simulink model "ClosedLoop_sim"  (Simulink 9.2)
settings: Solver=VariableStepAuto  StartTime=0.0  StopTime=10.0  RelTol=1e-3
libraries: neural x305, simulink x1
(part 13 of 13)

== system ClosedLoop_sim/bigger_controller/Layer 4/Delays 1 ==
  "p{4}" : Inport  PortDimensions=100
      mask Display: e = 0.06;c1 = [120 230 180]/255;c2 = ([120 230 180]+0)/(256+128);c3 = ([120 230 180]+128)/(256+128);patch([0 1 1 0],[0 0 1 1],c1);patch([0 1 1 1-e 1-e 0+e],[0 0 1 1-e 0+e 0+e],c2);patch([0 0 1 1-e 0+e 0+e],[0 1 1 1-e 1-e 0+e],c3);plot([0 1 1 0 0],[0 0 1 1 0]);
  mux : Mux  Inputs=1
      mask Display: e = 0.06;c1 = [120 150 230]/255;c2 = ([120 150 230]+0)/383;c3 = ([120 150 230]+128)/383;patch([0 1 1 0],[0 0 1 1],c1);patch([0 1 1 1-e 1-e 0+e],[0 0 1 1-e 0+e 0+e],c2);patch([0 0 1 1-e 0+e 0+e],[0 1 1 1-e 1-e 0+e],c3);plot([0 1 1 0 0],[0 0 1 1 0]);disp('Mux')
  "pd{4,3}" : Outport
      mask Display: e = 0.06;c1 = [120 230 180]/255;c2 = ([120 230 180]+0)/(256+128);c3 = ([120 230 180]+128)/(256+128);patch([0 1 1 0],[0 0 1 1],c1);patch([0 1 1 1-e 1-e 0+e],[0 0 1 1-e 0+e 0+e],c2);patch([0 0 1 1-e 0+e 0+e],[0 1 1 1-e 1-e 0+e],c3);plot([0 1 1 0 0],[0 0 1 1 0]);
  wires:
  mux/1 -> "pd{4,3}"/1
  "p{4}"/1 -> mux/1

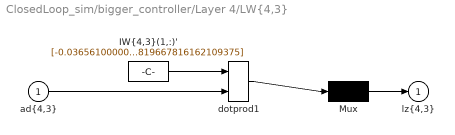
== system ClosedLoop_sim/bigger_controller/Layer 4/LW{4,3} ==
  "ad{4,3}" : Inport  PortDimensions=100
      mask Display: e = 0.06;c1 = [120 230 180]/255;c2 = ([120 230 180]+0)/(256+128);c3 = ([120 230 180]+128)/(256+128);patch([0 1 1 0],[0 0 1 1],c1);patch([0 1 1 1-e 1-e 0+e],[0 0 1 1-e 0+e 0+e],c2);patch([0 0 1 1-e 0+e 0+e],[0 1 1 1-e 1-e 0+e],c3);plot([0 1 1 0 0],[0 0 1 1 0]);
  "IW{4,3}(1,:)'" : Constant  Value=[-0.036561000000000003218314503783403779380023479461669921875;-0.09285100000000000297628588441511965356767177581787109375;-0.0752049999999999940758499406001647002995014190673828125;-0.01078299999999999918276483157342227059416472911834716796875;0.1605930000000000135162991909965057857334613800048828125;-0.06917700000000000237765362953723524697124958038330078125;0.311236000000000012644107982850982807576656341552734375;0.1429970000000000129869448528552311472594738006591796875;0.1426739999999999952695617366771330125629901885986328125;0.18814900000000001067945731847430579364299774169921875;0.14923100000000000253663756666355766355991363525390625;-0.1501159999999999994368948819101206026971340179443359375;0.06925199999999999411759432632607058621942996978759765625;-0.045718000000000001692423978738588630221784114837646484375;-0.0869270000000000042650327714000013656914234161376953125;0.0302669999999999987660981304316010209731757640838623046875;0.010054000000000000436539693282611551694571971893310546875;-0.083737000000000005872635711057228036224842071533203125;0.0338320000000000009610090501155355013906955718994140625;0.0203340000000000013791190411893694545142352581024169921875;-0.071068999999999993288923860745853744447231292724609375;-0.100376999999999994006572023863554932177066802978515625;0.039612000000000001376232461325344047509133815765380859375;0.054376000000000000722533144426051876507699489593505859375;0.1535060000000000035580427493187016807496547698974609375;-0.1376380000000000103366204484700574539601802825927734375;0.0712990000000000012647660696529783308506011962890625;-0.06631700000000000094768637382003362290561199188232421875;-0.0776840000000000030500046932502300478518009185791015625;0.1355139999999999955715423993751755915582180023193359375;0.09379999999999999449329379785922355949878692626953125;0.202359000000000011088019391536363400518894195556640625;-0.03459399999999999975042186406426480971276760101318359375;0.305327999999999988300913855709950439631938934326171875;0.1351590000000000013624656958199921064078807830810546875;0.1567389999999999894431113034443114884197711944580078125;-0.2571849999999999969446662362315692007541656494140625;0.06393400000000000471533923018796485848724842071533203125;0.1426429999999999920223814342534751631319522857666015625;-0.08723599999999999410338347161086858250200748443603515625;0.09323299999999999643218728806459694169461727142333984375;0.165463999999999999968025576890795491635799407958984375;0.2063480000000000036397551639311132021248340606689453125;0.07875300000000000355537821405960130505263805389404296875;-0.1585479999999999944915174410198233090341091156005859375;0.208137999999999989686472190442145802080631256103515625;-0.08697399999999999575805986751220189034938812255859375;-0.0752980000000000038173908478711382485926151275634765625;-0.08728700000000000347455397786688990890979766845703125;-0.0445959999999999967545960544157424010336399078369140625;-0.0831699999999999939337413934481446631252765655517578125;-0.1769779999999999964277463959660963155329227447509765625;-0.1027949999999999974864550722486455924808979034423828125;-0.14523900000000000698463509252178482711315155029296875;0.2129560000000000064002136923591024242341518402099609375;-0.0924709999999999976427744741158676333725452423095703125;-0.1609859999999999902176028854228206910192966461181640625;-0.04821999999999999897415392524635535664856433868408203125;0.138633000000000006224354365258477628231048583984375;0.084697999999999995512922623674967326223850250244140625;-0.1844490000000000018420820424580597318708896636962890625;-0.039683999999999997054800360274384729564189910888671875;-0.06112700000000000077893247407700982876121997833251953125;-0.11747100000000000596944715880454168654978275299072265625;-0.1331070000000000030926372573958360590040683746337890625;0.11905200000000000504218888863761094398796558380126953125;-0.1476200000000000012168044349891715683043003082275390625;-0.2219700000000000006394884621840901672840118408203125 ...(+1874 chars)]
      mask Display: e = 0.06;c1 = [120 150 230]/255;c2 = ([120 150 230]+0)/383;c3 = ([120 150 230]+128)/383;patch([0 1 1 0],[0 0 1 1],c1);patch([0 1 1 1-e 1-e 0+e],[0 0 1 1-e 0+e 0+e],c2);patch([0 0 1 1-e 0+e 0+e],[0 1 1 1-e 1-e 0+e],c3);plot([0 1 1 0 0],[0 0 1 1 0]);disp('weights');
  Mux : Mux  Inputs=1
      mask Display: e = 0.06;c1 = [120 150 230]/255;c2 = ([120 150 230]+0)/383;c3 = ([120 150 230]+128)/383;patch([0 1 1 0],[0 0 1 1],c1);patch([0 1 1 1-e 1-e 0+e],[0 0 1 1-e 0+e 0+e],c2);patch([0 0 1 1-e 0+e 0+e],[0 1 1 1-e 1-e 0+e],c3);plot([0 1 1 0 0],[0 0 1 1 0]);disp('Mux');
  dotprod1 : neural/Weight Functions/dotprod
  "lz{4,3}" : Outport
      mask Display: e = 0.06;c1 = [120 230 180]/255;c2 = ([120 230 180]+0)/(256+128);c3 = ([120 230 180]+128)/(256+128);patch([0 1 1 0],[0 0 1 1],c1);patch([0 1 1 1-e 1-e 0+e],[0 0 1 1-e 0+e 0+e],c2);patch([0 0 1 1-e 0+e 0+e],[0 1 1 1-e 1-e 0+e],c3);plot([0 1 1 0 0],[0 0 1 1 0]);
  wires:
  Mux/1 -> "lz{4,3}"/1
  dotprod1/1 -> Mux/1
  "ad{4,3}"/1 -> dotprod1/2
  "IW{4,3}(1,:)'"/1 -> dotprod1/1

== stateflow chart TORA ==
  settings: updateMethod=CONTINUOUS
  state TORA
    du:
    x1_dot = x2;
    x2_dot = -x1 + 0.1*sin(x3);
    x3_dot = x4;
    x4_dot = u;
    %OUTPUTS
    x1_out = x1;
    x2_out = x2;
    x3_out = x3;
    x4_out = x4;
  (default) -> TORA : {x1 = 0.65;
      | x2 = -0.65;
      | x3 = -0.35;
      | x4 = 0.55;}
  data: u input double; x1_out output double; x2_out output double; x3_out output double; x4_out output double; x1 local double; x2 local double; x3 local double; x4 local double
  data x1 settings: updateMethod=SF_CONTINUOUS_TIME_DATA
  data x2 settings: updateMethod=SF_CONTINUOUS_TIME_DATA
  data x3 settings: updateMethod=SF_CONTINUOUS_TIME_DATA
  data x4 settings: updateMethod=SF_CONTINUOUS_TIME_DATA
